simulink model "TC_Uno_OnOff_Control"  (R2018b)
settings: Solver=ode2  StartTime=0.0  StopTime=inf  FixedStep=1e-2  RelTol=1e-3  EnableMultiTasking=on
libraries: arduinolib x2
settings Model: SimulationMode=external  ExtModeTrigDuration=2  Creator=user  LastModifiedBy=auralius
settings OptimizationCC: EnhancedBackFolding=on  PassReuseOutputArgsAs=Individual arguments  MaxStackSize=64  OptimizeBlockOrder=speed  DifferentSizesBufferReuse=on  OptimizationCustomize=off
settings DebuggingCC: ParameterTunabilityLossMsg=error  LibraryContextMissingDiagnostic=none
settings HardwareCC: ProdBitPerInt=16  ProdBitPerPointer=16  ProdBitPerSizeT=16  ProdBitPerPtrDiffT=16  ProdLargestAtomicFloat=None  ProdWordSize=8  ProdHWDeviceType=Atmel->AVR
settings SFSimCC: SimCustomTerminator=analogWrite(9, 0);  SimUseLocalCustomCode=off  MATLABDynamicMemAlloc=off
settings RTWCC: SystemTargetFile=ert.tlc  HardwareBoard=Arduino Uno  TemplateMakefile=ert_default_tmf  GenerateReport=on  RTWUseLocalCustomCode=off  Toolchain=Arduino AVR  BuildConfiguration=Faster Runs  IncludeHyperlinkInReport=on  LaunchReport=on  GenerateTraceInfo=on  GenerateTraceReport=on  GenerateTraceReportSl=on  GenerateTraceReportSf=on  GenerateTraceReportEml=on
settings CodeAppCC: ForceParamTrailComments=on  IgnoreCustomStorageClasses=off  OperatorAnnotations=on  SimulinkDataObjDesc=on  SFDataObjDesc=on  InsertBlockDesc=on
settings ERTTargetCC: SupportContinuousTime=on  SupportVariableSizeSignals=on  ExtMode=on  ExtModeMexArgs='127.0.0.1' 0 17725

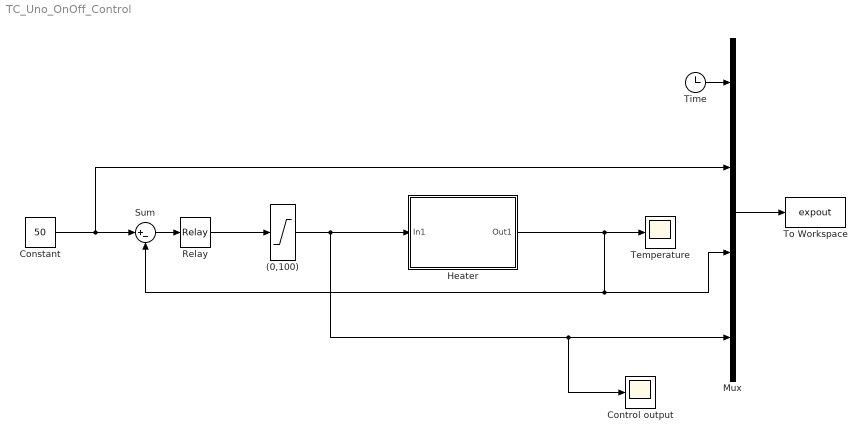
== system TC_Uno_OnOff_Control ==
  (0,100) : Saturate  UpperLimit=100  LowerLimit=0
  Constant : Constant  Value=50
  Control output : Scope
  Heater : Subsystem
  Mux : Mux
  Relay : Relay  OnSwitchValue=1  OffSwitchValue=-1  OnOutputValue=100
  Sum : Sum  Inputs=|+-
  Temperature : Scope
  Time : Clock
  To Workspace : ToWorkspace  VariableName=expout  SampleTime=-1
  wires:
  Mux/1 -> To Workspace/1
  Relay/1 -> (0,100)/1
  Time/1 -> Mux/1
  Heater/1(Out1) -> Sum/2, Mux/3, Temperature/1
  (0,100)/1 -> Control output/1, Mux/4, Heater/1(In1)
  Constant/1 -> Mux/2, Sum/1
  Sum/1 -> Relay/1

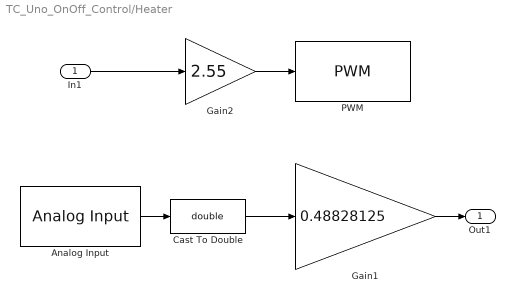
== system TC_Uno_OnOff_Control/Heater ==
  In1 : Inport
  Analog Input : arduinolib/Analog Input  pinNumber=0  ReadResultsOnly=off  ConversionTriggerSource=Software  ExternalTriggerType=uint32(0)  OutputDataType=uint16  EnableConversionCompleteNotify=off  EnableOuputStatus=off  SampleTime=-1  blockPlatform=arduino
  Cast To Double : DataTypeConversion  OutDataTypeStr=double
  Gain1 : Gain  Gain=0.48828125
  Gain2 : Gain  Gain=2.55
  PWM : arduinolib/PWM  pinNumber=9  EnableInputFrequency=off  InitialFrequency=2000  InitialDutyCycle=0  NotificationType=None  blockPlatform=arduino
  Out1 : Outport
  wires:
  Gain1/1 -> Out1/1
  In1/1 -> Gain2/1
  Gain2/1 -> PWM/1
  Analog Input/1 -> Cast To Double/1
  Cast To Double/1 -> Gain1/1
